simulink model "final_VVVF_control"  (R2018b)
settings: Solver=ode23t  StartTime=0.0  StopTime=3  RelTol=1e-3
undefined symbols (not defined in the file): Ts
libraries: powerlib x23, simulink x6, powerlib_meascontrol x4
settings Model: Creator=13646769405  LastModifiedBy=13646769405

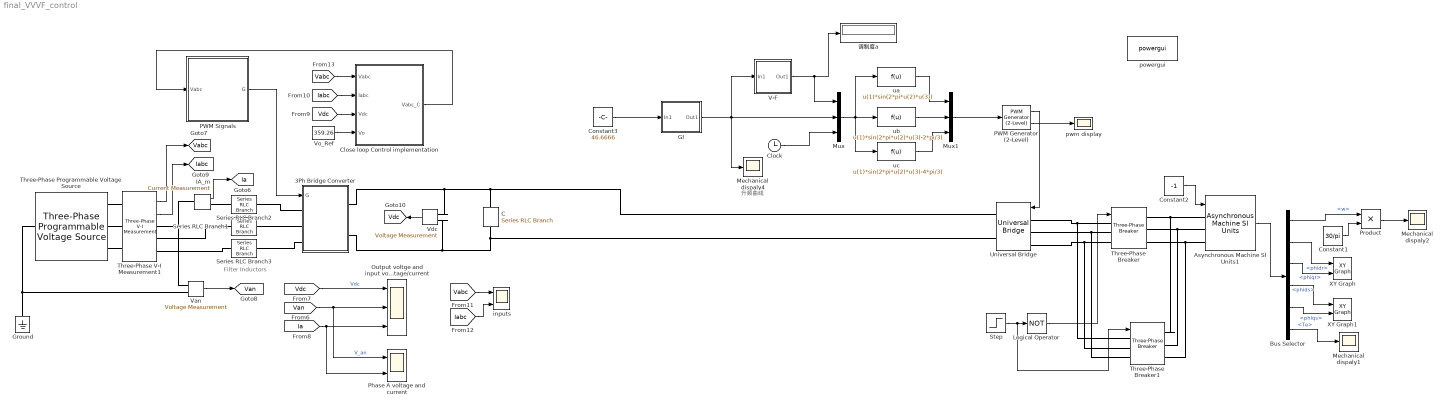
== system final_VVVF_control ==
  note: 升频曲线
  note: Filter Inductors
  3Ph Bridge Converter : Subsystem
  Asynchronous Machine SI Units1 : powerlib/Machines/Asynchronous Machine SI Units  RotorType=Squirrel-cage  PresetModel=No  MechanicalLoad=Torque Tm  ShowDetailedParameters=on  ReferenceFrame=Stationary  Units=SI  MeasurementBus=on  NominalParameters=[ 3*746, 220, 60 ]  Stator=[ 0.435 2*2.0e-3 ]  Rotor=[ 0.816 2.0e-3 ]  Cage1=[ 0.022 0.226/377]  Cage2=[ 0.022 0.226/377]  Lm=69.31e-3  Mechanical="[ 0.089  0  2 ]"  PolePairs=2  InitialConditions=[1 0 0 0 0 0 0 0]  SimulateSaturation=off  Saturation=[14.03593122, 27.81365428, 53.79336849, 72.68890987, 97.98006896, 148.6815601, 215.7428561, 302.9841135, 420.4778367 ; 230, 322, 414, 460, 506, 552, 598, 644, 690]  LoadFlowParameters=1492000  TsPowergui=0  TsBlock=-1  IterativeModel=Forward Euler  IterativeDiscreteModel=Trapezoidal non iterative  Pmec=0
  Bus Selector : BusSelector  OutputSignals=w,phidr,phiqr,phids,phiqs,Te
  C : powerlib/Elements/Series RLC Branch  LConnTagsString=__new0  RConnTagsString=__new0  BranchType=C  Resistance=1  Inductance=1e-3  SetiL0=off  InitialCurrent=0  Capacitance=1000e-6  Setx0=off  InitialVoltage=0  Measurements=None
      settings: SourceProductName=Simscape Electrical
  Clock : Clock
  Close loop Control implementation : Subsystem
  Constant1 : Constant  Value=30/pi
  Constant2 : Constant  Value=-1
  Constant3 : Constant  Value=46.6666
  GI : Subsystem
  Ground : powerlib/Elements/Ground  LConnTagsString=a
      settings: SourceProductName=Simscape Electrical
  IA_m : powerlib/Measurements/Current Measurement  PhasorSimulation=off  OutputType=Complex  PSBequivalent=0
      settings: SourceProductName=Simscape Electrical
  Logical Operator : Logic  Operator=NOT  AllPortsSameDT=off  OutDataTypeStr=boolean
  Mechanical dispaly1 : Scope
  Mechanical dispaly2 : Scope
  Mechanical dispaly4 : Scope
  Mux : Mux  Inputs=3
  Mux1 : Mux  Inputs=3
  Output voltge and input voltage/current : Scope  NumInputPorts=3
  PWM Generator (2-Level) : powerlib_meascontrol/Pulse & Signal Generators/PWM Generator (2-Level)  ModulatorType=Three-phase bridge (6 pulses)  ModulatorMode=Unsynchronized  Fc=1000  Pc=0  nF=27  MinMax="[ -1  1 ]"  SamplingTechnique=Natural  ModulatingSignals=off  m=1  Freq=40  Phase=0  Ts=0  ShowCarrierOutport=on
  PWM Signals : Subsystem
  Phase A voltage and current : Scope  NumInputPorts=2
  Product : Product
  Series RLC Branch1 : powerlib/Elements/Series RLC Branch  LConnTagsString=__new0  RConnTagsString=__new0  BranchType=RL  Resistance=.1  Inductance=1e-3  SetiL0=off  InitialCurrent=0  Capacitance=200e-6  Setx0=off  InitialVoltage=0  Measurements=None
      settings: SourceProductName=Simscape Electrical
  Series RLC Branch2 : powerlib/Elements/Series RLC Branch  LConnTagsString=__new0  RConnTagsString=__new0  BranchType=RL  Resistance=0.1  Inductance=1e-3  SetiL0=off  InitialCurrent=0  Capacitance=200e-6  Setx0=off  InitialVoltage=0  Measurements=None
      settings: SourceProductName=Simscape Electrical
  Series RLC Branch3 : powerlib/Elements/Series RLC Branch  LConnTagsString=__new0  RConnTagsString=__new0  BranchType=RL  Resistance=0.1  Inductance=1e-3  SetiL0=off  InitialCurrent=0  Capacitance=200e-6  Setx0=off  InitialVoltage=0  Measurements=None
      settings: SourceProductName=Simscape Electrical
  Step : Step  Time=3  Before=1  SampleTime=0
  Three-Phase Programmable Voltage Source : powerlib/Electrical Sources/Three-Phase Programmable Voltage Source  PositiveSequence="[220*1.732  0 60]"  VariationEntity=None  VariationType=Table of time-amplitude pairs  VariationTypeAlt=Step  VariationStep=0.5  VariationRate=10  VariationMagnitude=0.3  VariationFrequency=2  VariationTiming=[1 2]  VariationPhaseA=off  Amplitudes=[1 0.8 1.2 1.0]  TimeValues=[0 0.1 0.15 0.2]  HarmonicGeneration=on  HarmonicA=[3 0.2 -25 0]  HarmonicB=[2 0.15 35 2]  Timing="[0.05  3]"  BusType=swing  Pref=0  Qref=0  Qmin=-inf  Qmax=inf
      settings: SourceProductName=Simscape Electrical
  Three-Phase V-I Measurement1 : powerlib/Measurements/Three-Phase V-I Measurement  VoltageMeasurement=phase-to-ground  SetLabelV=off  LabelV=Vabc  Vpu=off  VpuLL=off  CurrentMeasurement=yes  SetLabelI=off  LabelI=Iabc  Ipu=off  Pbase=100e6  Vbase=500e3  OutputType=Complex  PhasorSimulation=off  PSBequivalent=0
      settings: SourceProductName=Simscape Electrical
  Three-Phase Breaker : powerlib/Elements/Three-Phase Breaker  InitialState=open  SwitchA=on  SwitchB=on  SwitchC=on  SwitchTimes="[1/60  5/60]"  External=on  BreakerResistance=0.01  SnubberResistance=1e6  SnubberCapacitance=inf  Measurements=None
      settings: SourceProductName=Simscape Electrical
  Three-Phase Breaker1 : powerlib/Elements/Three-Phase Breaker  InitialState=open  SwitchA=on  SwitchB=on  SwitchC=on  SwitchTimes="[1/60  5/60]"  External=on  BreakerResistance=0.01  SnubberResistance=1e6  SnubberCapacitance=inf  Measurements=None
      settings: SourceProductName=Simscape Electrical
  Universal Bridge : powerlib/Power Electronics/Universal Bridge  Arms=3  SnubberResistance=1e5  SnubberCapacitance=inf  Device=IGBT / Diodes  Ron=1e-3  Lon=0  ForwardVoltages="[  0  0  ]"  ForwardVoltage=0  GTOparameters=[ 10e-6 , 20e-6 ]  IGBTparameters=[ 1e-6 , 2e-6 ]  Measurements=None  Measurements_2=None  converterType=Rectifier
      settings: SourceProductName=Simscape Electrical
  V-F : Subsystem
  Van : powerlib/Measurements/Voltage Measurement  Tag=PoWeRsYsTeMmEaSuReMeNt  PhasorSimulation=off  OutputType=Magnitude  PSBequivalent=0
      settings: SourceProductName=Simscape Electrical
  "Vdc " : powerlib/Measurements/Voltage Measurement  Tag=PoWeRsYsTeMmEaSuReMeNt  PhasorSimulation=off  OutputType=Magnitude  PSBequivalent=0
      settings: SourceProductName=Simscape Electrical
  Vo_Ref : Constant  Value=359.26
  XY Graph : simulink/Sinks/XY Graph  xmin=-1  xmax=1  ymin=-1  ymax=1  st=-1
  XY Graph1 : simulink/Sinks/XY Graph  xmin=-1  xmax=1  ymin=-1  ymax=1  st=-1
  inputs : Scope  NumInputPorts=2
  powergui : powerlib/powergui  Priority=1  SimulationMode=Discrete  SampleTime=1e-5  frequency=60  Iterations=50  frequencyindice=60  Pbase=100e6  ErrMax=1e-4  UnitsV=kV  UnitsW=MW  buscounter=0  FunctionMessages=off  echomessages=off  EnableUseOfTLC=off  CurrentSourceSwitches=off  DisableSnubberDevices=off  DisableRonSwitches=off  DisableVfSwitches=off  DisplayEquations=off  SolverType=Tustin/Backward Euler (TBE)  Interpol=off  ExternalGateDelay=off  methode=off  Ts=100  x0status=blocks  SPID=on  SwTol=0  HookPort=off  RestoreLinks=warning  ResistiveCurrentMeasurement=off  Frange=[0:2:500]  Ylog=off  Xlog=on  ShowGrid=off  save=off  variable=ZData  structure=0  ZoomFFT=off  StartTime=0.0  cycles=1  DisplayStyle=1  fundamental=60  FreqAxis=off  MaxFrequency=1000  frequencyindicesteady=1  RmsSteady=1  display=off
  pwm display : Scope
  ua : Fcn  Expr=u(1)*sin(2*pi*u(2)*u(3))
  ub : Fcn  Expr=u(1)*sin(2*pi*u(2)*u(3)-2*pi/3)
  uc : Fcn  Expr=u(1)*sin(2*pi*u(2)*u(3)-4*pi/3)
  调制度a : Display
  tag scope: Ia=global, Iabc=global, Vabc=global, Van=global, Vdc=global
  wires:
  Constant1/1 -> Product/2
  Product/1 -> Mechanical dispaly2/1
  Bus Selector/1 -> Product/1  "<w>"
  Mux1/1 -> PWM Generator (2-Level)/1
  ub/1 -> Mux1/2
  uc/1 -> Mux1/3
  ua/1 -> Mux1/1
  Clock/1 -> Mux/3
  Mux/1 -> ua/1, uc/1, ub/1
  PWM Generator (2-Level)/1 -> Universal Bridge/1
  PWM Generator (2-Level)/2 -> pwm display/1
  GI/1(Out1) -> Mechanical dispaly4/1, Mux/2, V-F/1(In1)
  V-F/1(Out1) -> Mux/1, 调制度a/1
  Constant2/1 -> Asynchronous Machine SI Units1/1
  Constant3/1 -> GI/1(In1)
  Asynchronous Machine SI Units1/1 -> Bus Selector/1
  Step/1 -> Three-Phase Breaker1/1, Logical Operator/1
  Logical Operator/1 -> Three-Phase Breaker/1
  PWM Signals/1(G) -> 3Ph Bridge Converter/1(G)
  Three-Phase V-I Measurement1/1 -> [Vabc]
  [Vabc] -> inputs/1
  Three-Phase V-I Measurement1/2 -> [Iabc]
  [Ia] -> Phase A voltage and current/2, Output voltge and input voltage/current/3
  [Van] -> Phase A voltage and current/1, Output voltge and input voltage/current/2  "V_an"
  [Vdc] -> Output voltge and input voltage/current/1  "Vdc"
  IA_m/1 -> [Ia]
  [Vabc] -> Close loop Control implementation/1(Vabc)
  [Iabc] -> inputs/2
  [Vdc] -> Close loop Control implementation/3(Vdc)
  Vo_Ref/1 -> Close loop Control implementation/4(Vo)
  Van/1 -> [Van]
  "Vdc "/1 -> [Vdc]
  Close loop Control implementation/1(Vabc_C) -> PWM Signals/1(Vabc)
  [Iabc] -> Close loop Control implementation/2(Iabc)
  Bus Selector/2 -> XY Graph/1  "<phidr>"
  Bus Selector/3 -> XY Graph/2  "<phiqr>"
  Bus Selector/4 -> XY Graph1/1  "<phids>"
  Bus Selector/5 -> XY Graph1/2  "<phiqs>"
  Bus Selector/6 -> Mechanical dispaly1/1  "<Te>"
  connections:
  3Ph Bridge Converter/RConn1 -- Universal Bridge/RConn1 -- C/LConn1 -- "Vdc "/LConn1
  Three-Phase Breaker/LConn1 -- Three-Phase Breaker1/LConn1 -- Universal Bridge/LConn1
  Three-Phase Breaker/LConn3 -- Three-Phase Breaker1/LConn2 -- Universal Bridge/LConn3
  Three-Phase Breaker/RConn1 -- Asynchronous Machine SI Units1/LConn1 -- Three-Phase Breaker1/RConn1
  Three-Phase Breaker/RConn2 -- Three-Phase Breaker1/RConn2 -- Asynchronous Machine SI Units1/LConn2
  Asynchronous Machine SI Units1/LConn3 -- Three-Phase Breaker1/RConn3 -- Three-Phase Breaker/RConn3
  Three-Phase V-I Measurement1/RConn1 -- Van/LConn1 -- IA_m/LConn1
  "Vdc "/LConn2 -- Universal Bridge/RConn2 -- C/RConn1 -- 3Ph Bridge Converter/RConn2
  Three-Phase Programmable Voltage Source/LConn1 -- Ground/LConn1 -- Van/LConn2
  Three-Phase V-I Measurement1/RConn3 -- Series RLC Branch3/RConn1
  Three-Phase V-I Measurement1/RConn2 -- Series RLC Branch1/RConn1
  Three-Phase V-I Measurement1/LConn2 -- Three-Phase Programmable Voltage Source/RConn2
  Series RLC Branch3/LConn1 -- 3Ph Bridge Converter/LConn3
  Series RLC Branch2/LConn1 -- 3Ph Bridge Converter/LConn1
  Three-Phase V-I Measurement1/LConn3 -- Three-Phase Programmable Voltage Source/RConn3
  Three-Phase V-I Measurement1/LConn1 -- Three-Phase Programmable Voltage Source/RConn1
  Series RLC Branch1/LConn1 -- 3Ph Bridge Converter/LConn2
  IA_m/RConn1 -- Series RLC Branch2/RConn1
  Universal Bridge/LConn2 -- Three-Phase Breaker1/LConn3 -- Three-Phase Breaker/LConn2

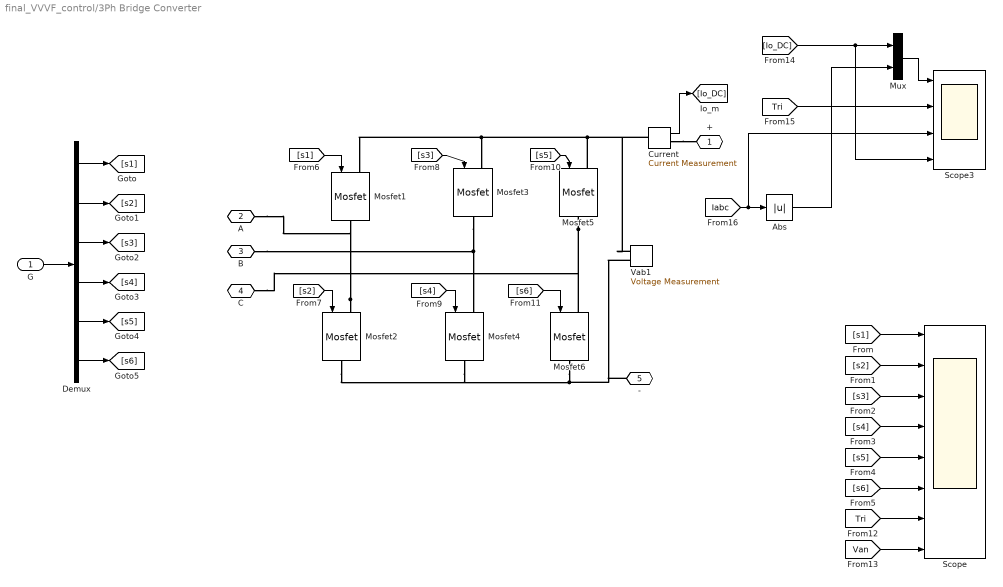
== system final_VVVF_control/3Ph Bridge Converter ==
  G : Inport
  Abs : Abs
  Current : powerlib/Measurements/Current Measurement  PhasorSimulation=off  OutputType=Complex  PSBequivalent=0
      settings: SourceProductName=Simscape Electrical
  Demux : Demux  Outputs=6
  Mosfet{1..6} (6 alike) : powerlib/Power Electronics/Mosfet  Ron=0.1  Lon=0  Rd=0.01  Vfd=0  IC=0  Rs=1e5  Cs=inf  Measurements=off
      settings: SourceProductName=Simscape Electrical
  Mux : Mux  Inputs=2
  Scope : Scope  NumInputPorts=8
  Scope3 : Scope  NumInputPorts=4
  Vab1 : powerlib/Measurements/Voltage Measurement  Tag=PoWeRsYsTeMmEaSuReMeNt  PhasorSimulation=off  OutputType=Magnitude  PSBequivalent=0
      settings: SourceProductName=Simscape Electrical
  + : PMIOPort  Side=Right
  A : PMIOPort  Port=2  Side=Left
  B : PMIOPort  Port=3  Side=Left
  C : PMIOPort  Port=4  Side=Left
  - : PMIOPort  Port=5  Side=Right
  wires:
  [s1] -> Mosfet1/1
  [s2] -> Mosfet2/1
  [s3] -> Mosfet3/1
  [s4] -> Mosfet4/1
  [s5] -> Mosfet5/1
  [s6] -> Mosfet6/1
  Demux/1 -> [s1]
  Demux/2 -> [s2]
  Demux/3 -> [s3]
  Demux/4 -> [s4]
  Demux/5 -> [s5]
  Demux/6 -> [s6]
  G/1 -> Demux/1
  Current/1 -> [Io_DC]
  [s1] -> Scope/1
  [s2] -> Scope/2
  [s3] -> Scope/3
  [s4] -> Scope/4
  [s5] -> Scope/5
  [s6] -> Scope/6
  [Tri] -> Scope/7
  [Van] -> Scope/8
  [Tri] -> Scope3/2
  [Io_DC] -> Scope3/4, Mux/1
  Mux/1 -> Scope3/1
  [Iabc] -> Scope3/3, Abs/1
  Abs/1 -> Mux/2
  connections:
  Mosfet5/LConn1 -- Vab1/LConn1 -- Current/LConn1 -- Mosfet1/LConn1 -- Mosfet3/LConn1
  Mosfet6/RConn1 -- Vab1/LConn2 -- -/RConn1 -- Mosfet2/RConn1 -- Mosfet4/RConn1
  Mosfet2/LConn1 -- Mosfet1/RConn1 -- A/RConn1
  Mosfet3/RConn1 -- Mosfet4/LConn1 -- B/RConn1
  Mosfet5/RConn1 -- Mosfet6/LConn1 -- C/RConn1
  Current/RConn1 -- +/RConn1

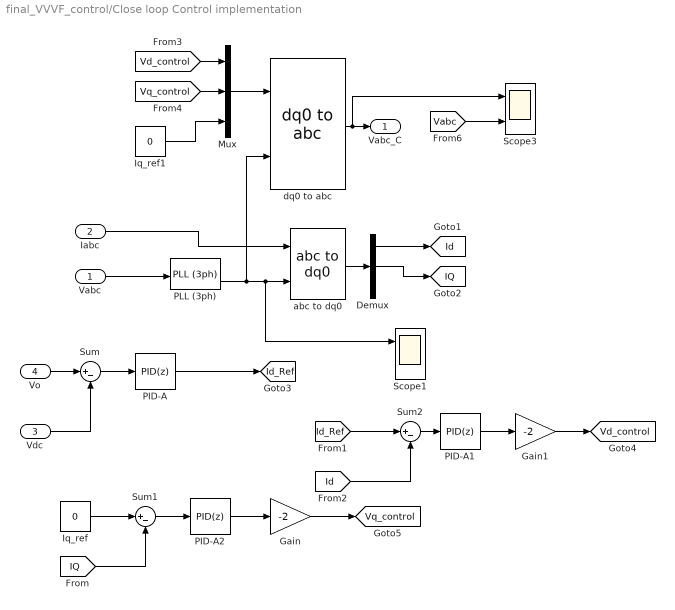
== system final_VVVF_control/Close loop Control implementation ==
  Vabc : Inport
  Iabc : Inport  Port=2
  Vdc : Inport  Port=3
  Vo : Inport  Port=4
  Demux : Demux  Outputs=3
  Gain : Gain  Gain=-2
  Gain1 : Gain  Gain=-2
  Iq_ref : Constant  Value=0
  Iq_ref1 : Constant  Value=0
  Mux : Mux  Inputs=3
  PID-A : simulink/Continuous/PID Controller  Controller=PID  Form=Parallel  TimeDomain=Discrete-time  SampleTime=Ts  IntegratorMethod=Forward Euler  FilterMethod=Forward Euler  ControllerParametersSource=internal  P=0.2  I=0.2/0.002  D=0  UseFilter=on  N=100  TunerSelectOption=Transfer Function Based (PID Tuner App)  InitialConditionSource=internal  InitialConditionForIntegrator=0  InitialConditionForFilter=0  DifferentiatorICPrevScaledInput=0  ExternalReset=none  TrackingMode=off  Kt=1  LimitOutput=off  UpperSaturationLimit=inf  LowerSaturationLimit=-inf  LinearizeAsGain=on  AntiWindupMode=none  Kb=1  POutMin=[]  POutMax=[]  IOutMin=[]  IOutMax=[]  DOutMin=[]  DOutMax=[]  NOutMin=[]  NOutMax=[]  SumOutMin=[]  SumOutMax=[]  SaturationOutMin=[]  SaturationOutMax=[]  PParamMin=[]  PParamMax=[]  IParamMin=[]  IParamMax=[]  DParamMin=[]  DParamMax=[]  NParamMin=[]  NParamMax=[]  KbParamMin=[]  KbParamMax=[]  KtParamMin=[]  KtParamMax=[]  KbOutMin=[]  KbOutMax=[]  KtOutMin=[]  KtOutMax=[]  IntegratorOutMin=[]  IntegratorOutMax=[]  FilterOutMin=[]  FilterOutMax=[]  SumI1OutMin=[]  SumI1OutMax=[]  SumI2OutMin=[]  SumI2OutMax=[]  SumI3OutMin=[]  SumI3OutMax=[]  SumI4OutMin=[]  SumI4OutMax=[]  SumDOutMin=[]  SumDOutMax=[]  DifferentiatorOutMin=[]  DifferentiatorOutMax=[]  FilterDiffOutCoefMin=[]  FilterDiffOutCoefMax=[]  ReciprocalOutMin=[]  ReciprocalOutMax=[]  SumDenOutMin=[]  SumDenOutMax=[]  SumNumOutMin=[]  SumNumOutMax=[]  DivideOutMin=[]  DivideOutMax=[]  IntegratorContinuousStateAttributes=''  IntegratorStateMustResolveToSignalObject=off  IntegratorRTWStateStorageClass=Auto  FilterContinuousStateAttributes=''  FilterStateMustResolveToSignalObject=off  FilterRTWStateStorageClass=Auto  ParallelPVariant=InternalParameters  IdealPVariant=Disabled  IVariant=InternalParameters  DVariant=InternalParameters  IntegratorVariant=Discrete  SatVariant=Disabled  AWVariant=Passthrough  PCopyVariant=Disabled  TRVariant=Disabled  FdbkBlocksVariant=Forward  IdealPFdbkVariant=Disabled  SatFdbkVariant=Disabled  DerivativeFilterVariant=ForwardEulerFilter  NVariant=InternalParameters  NCopyVariant=Disabled  FilterICVariant=InternalICsFilter  IntegratorICVariant=InternalICs  ExternalResetVariant=Disabled  TRSumVariant=Passthrough  SumFdbkVariant=Disabled  SumVariant=Sum_PID
  PID-A1 : simulink/Continuous/PID Controller  Controller=PID  Form=Parallel  TimeDomain=Discrete-time  SampleTime=-1  IntegratorMethod=Forward Euler  FilterMethod=Forward Euler  ControllerParametersSource=internal  P=6.225/270  I=0.0231/1.172e-3  D=0  UseFilter=on  N=100  TunerSelectOption=Transfer Function Based (PID Tuner App)  InitialConditionSource=internal  InitialConditionForIntegrator=0  InitialConditionForFilter=0  DifferentiatorICPrevScaledInput=0  ExternalReset=none  TrackingMode=off  Kt=1  LimitOutput=off  UpperSaturationLimit=inf  LowerSaturationLimit=-inf  LinearizeAsGain=on  AntiWindupMode=none  Kb=1  POutMin=[]  POutMax=[]  IOutMin=[]  IOutMax=[]  DOutMin=[]  DOutMax=[]  NOutMin=[]  NOutMax=[]  SumOutMin=[]  SumOutMax=[]  SaturationOutMin=[]  SaturationOutMax=[]  PParamMin=[]  PParamMax=[]  IParamMin=[]  IParamMax=[]  DParamMin=[]  DParamMax=[]  NParamMin=[]  NParamMax=[]  KbParamMin=[]  KbParamMax=[]  KtParamMin=[]  KtParamMax=[]  KbOutMin=[]  KbOutMax=[]  KtOutMin=[]  KtOutMax=[]  IntegratorOutMin=[]  IntegratorOutMax=[]  FilterOutMin=[]  FilterOutMax=[]  SumI1OutMin=[]  SumI1OutMax=[]  SumI2OutMin=[]  SumI2OutMax=[]  SumI3OutMin=[]  SumI3OutMax=[]  SumI4OutMin=[]  SumI4OutMax=[]  SumDOutMin=[]  SumDOutMax=[]  DifferentiatorOutMin=[]  DifferentiatorOutMax=[]  FilterDiffOutCoefMin=[]  FilterDiffOutCoefMax=[]  ReciprocalOutMin=[]  ReciprocalOutMax=[]  SumDenOutMin=[]  SumDenOutMax=[]  SumNumOutMin=[]  SumNumOutMax=[]  DivideOutMin=[]  DivideOutMax=[]  IntegratorContinuousStateAttributes=''  IntegratorStateMustResolveToSignalObject=off  IntegratorRTWStateStorageClass=Auto  FilterContinuousStateAttributes=''  FilterStateMustResolveToSignalObject=off  FilterRTWStateStorageClass=Auto  ParallelPVariant=InternalParameters  IdealPVariant=Disabled  IVariant=InternalParameters  DVariant=InternalParameters  IntegratorVariant=Discrete  SatVariant=Disabled  AWVariant=Passthrough  PCopyVariant=Disabled  TRVariant=Disabled  FdbkBlocksVariant=Forward  IdealPFdbkVariant=Disabled  SatFdbkVariant=Disabled  DerivativeFilterVariant=ForwardEulerFilter  NVariant=InternalParameters  NCopyVariant=Disabled  FilterICVariant=InternalICsFilter  IntegratorICVariant=InternalICs  ExternalResetVariant=Disabled  TRSumVariant=Passthrough  SumFdbkVariant=Disabled  SumVariant=Sum_PID
  PID-A2 : simulink/Continuous/PID Controller  Controller=PID  Form=Parallel  TimeDomain=Discrete-time  SampleTime=-1  IntegratorMethod=Forward Euler  FilterMethod=Forward Euler  ControllerParametersSource=internal  P=6.225/270  I=0.0231/1.172e-3  D=0  UseFilter=on  N=100  TunerSelectOption=Transfer Function Based (PID Tuner App)  InitialConditionSource=internal  InitialConditionForIntegrator=0  InitialConditionForFilter=0  DifferentiatorICPrevScaledInput=0  ExternalReset=none  TrackingMode=off  Kt=1  LimitOutput=off  UpperSaturationLimit=inf  LowerSaturationLimit=-inf  LinearizeAsGain=on  AntiWindupMode=none  Kb=1  POutMin=[]  POutMax=[]  IOutMin=[]  IOutMax=[]  DOutMin=[]  DOutMax=[]  NOutMin=[]  NOutMax=[]  SumOutMin=[]  SumOutMax=[]  SaturationOutMin=[]  SaturationOutMax=[]  PParamMin=[]  PParamMax=[]  IParamMin=[]  IParamMax=[]  DParamMin=[]  DParamMax=[]  NParamMin=[]  NParamMax=[]  KbParamMin=[]  KbParamMax=[]  KtParamMin=[]  KtParamMax=[]  KbOutMin=[]  KbOutMax=[]  KtOutMin=[]  KtOutMax=[]  IntegratorOutMin=[]  IntegratorOutMax=[]  FilterOutMin=[]  FilterOutMax=[]  SumI1OutMin=[]  SumI1OutMax=[]  SumI2OutMin=[]  SumI2OutMax=[]  SumI3OutMin=[]  SumI3OutMax=[]  SumI4OutMin=[]  SumI4OutMax=[]  SumDOutMin=[]  SumDOutMax=[]  DifferentiatorOutMin=[]  DifferentiatorOutMax=[]  FilterDiffOutCoefMin=[]  FilterDiffOutCoefMax=[]  ReciprocalOutMin=[]  ReciprocalOutMax=[]  SumDenOutMin=[]  SumDenOutMax=[]  SumNumOutMin=[]  SumNumOutMax=[]  DivideOutMin=[]  DivideOutMax=[]  IntegratorContinuousStateAttributes=''  IntegratorStateMustResolveToSignalObject=off  IntegratorRTWStateStorageClass=Auto  FilterContinuousStateAttributes=''  FilterStateMustResolveToSignalObject=off  FilterRTWStateStorageClass=Auto  ParallelPVariant=InternalParameters  IdealPVariant=Disabled  IVariant=InternalParameters  DVariant=InternalParameters  IntegratorVariant=Discrete  SatVariant=Disabled  AWVariant=Passthrough  PCopyVariant=Disabled  TRVariant=Disabled  FdbkBlocksVariant=Forward  IdealPFdbkVariant=Disabled  SatFdbkVariant=Disabled  DerivativeFilterVariant=ForwardEulerFilter  NVariant=InternalParameters  NCopyVariant=Disabled  FilterICVariant=InternalICsFilter  IntegratorICVariant=InternalICs  ExternalResetVariant=Disabled  TRSumVariant=Passthrough  SumFdbkVariant=Disabled  SumVariant=Sum_PID
  PLL (3ph) : powerlib_meascontrol/PLL/PLL (3ph)  Fmin=45  Par_Init=[0, 60]  ParK=[180, 3200, 1]  TcD=1e-4  MaxRateChangeFreq=12  FilterCutOffFreq=25  Ts=0  AGC=on
      settings: SourceProductName=Simscape Electrical
  Scope1 : Scope  NumInputPorts=2
  Scope3 : Scope  NumInputPorts=2
  Sum : Sum  Inputs=|+-
  Sum1 : Sum  Inputs=|+-
  Sum2 : Sum  Inputs=|+-
  abc to dq0 : powerlib_meascontrol/Transformations/abc to dq0  Alignment=90 degrees behind phase A axis
      settings: SourceProductName=Simscape Electrical
  dq0 to abc : powerlib_meascontrol/Transformations/dq0 to abc  Alignment=90 degrees behind phase A axis
      settings: SourceProductName=Simscape Electrical
  Vabc_C : Outport
  tag scope: IQ=global, Id=global, Id_Ref=global, Vd_control=global, Vq_control=global
  wires:
  Vabc/1 -> PLL (3ph)/1
  PLL (3ph)/2 -> dq0 to abc/2, Scope1/1, abc to dq0/2
  Iabc/1 -> abc to dq0/1
  abc to dq0/1 -> Demux/1
  Demux/1 -> [Id]
  Demux/2 -> [IQ]
  Iq_ref/1 -> Sum1/1
  [IQ] -> Sum1/2
  Sum1/1 -> PID-A2/1
  [Id_Ref] -> Sum2/1
  [Id] -> Sum2/2
  Sum2/1 -> PID-A1/1
  PID-A2/1 -> Gain/1
  PID-A1/1 -> Gain1/1
  Mux/1 -> dq0 to abc/1
  [Vd_control] -> Mux/1
  [Vq_control] -> Mux/2
  Iq_ref1/1 -> Mux/3
  dq0 to abc/1 -> Scope3/1, Vabc_C/1
  Gain/1 -> [Vq_control]
  Gain1/1 -> [Vd_control]
  [Vabc] -> Scope3/2
  Sum/1 -> PID-A/1
  Vo/1 -> Sum/1
  Vdc/1 -> Sum/2
  PID-A/1 -> [Id_Ref]

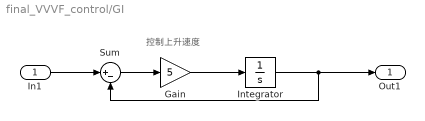
== system final_VVVF_control/GI ==
  note: 控制上升速度
  In1 : Inport
  Gain : Gain  Gain=5
  Integrator : Integrator
  Sum : Sum  Inputs=|+-
  Out1 : Outport
  wires:
  Integrator/1 -> Out1/1, Sum/2
  Gain/1 -> Integrator/1
  In1/1 -> Sum/1
  Sum/1 -> Gain/1

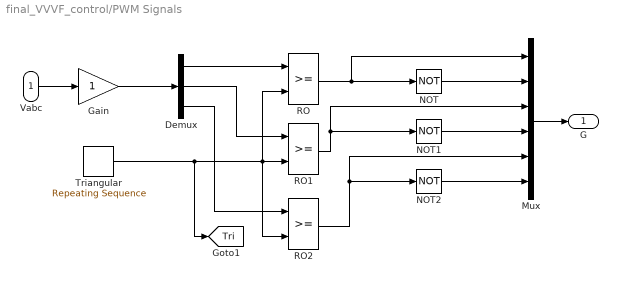
== system final_VVVF_control/PWM Signals ==
  Vabc : Inport
  Demux : Demux  Outputs=3
  Gain : Gain
  Mux : Mux  Inputs=6
  NOT : Logic  Operator=NOT  IconShape=distinctive  AllPortsSameDT=off  OutDataTypeStr=boolean
  NOT1 : Logic  Operator=NOT  IconShape=distinctive  AllPortsSameDT=off  OutDataTypeStr=boolean
  NOT2 : Logic  Operator=NOT  IconShape=distinctive  AllPortsSameDT=off  OutDataTypeStr=boolean
  RO : RelationalOperator  OutDataTypeStr=boolean  RndMeth=Nearest
  RO1 : RelationalOperator  OutDataTypeStr=boolean  RndMeth=Nearest
  RO2 : RelationalOperator  OutDataTypeStr=boolean  RndMeth=Nearest
  Triangular : simulink/Sources/Repeating Sequence  rep_seq_t="[0  1/(10e3) 1/(5e3) ]"  rep_seq_y=[-1 1 -1 ]
  G : Outport
  tag scope: Tri=global
  wires:
  Vabc/1 -> Gain/1
  Gain/1 -> Demux/1
  Demux/1 -> RO/1
  Demux/2 -> RO1/1
  Demux/3 -> RO2/1
  Triangular/1 -> [Tri], RO1/2, RO/2, RO2/2
  RO/1 -> Mux/1, NOT/1
  NOT/1 -> Mux/2
  RO2/1 -> NOT2/1, Mux/5
  RO1/1 -> NOT1/1, Mux/3
  NOT1/1 -> Mux/4
  NOT2/1 -> Mux/6
  Mux/1 -> G/1

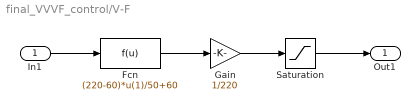
== system final_VVVF_control/V-F ==
  In1 : Inport
  Fcn : Fcn  Expr=(220-60)*u(1)/50+60
  Gain : Gain  Gain=1/220
  Saturation : Saturate  UpperLimit=0.95  LowerLimit=-0.95
  Out1 : Outport
  wires:
  Fcn/1 -> Gain/1
  In1/1 -> Fcn/1
  Gain/1 -> Saturation/1
  Saturation/1 -> Out1/1
